simulink model "gov_modularised"  (R2020a)
settings: Solver=VariableStepAuto  StartTime=0.0  StopTime=10.0  RelTol=1e-3
values from neighbouring files (symbols this model uses):
  Amp = 0.1*10^6    (= 100000)    [main.m]
  Kd = 0.2*10^6    (= 200000)    [main.m]
  Ki = 0.2*10^6    (= 200000)    [main.m]
  Kp = 1*10^6    (= 1000000)    [main.m]
  sigma = 0.6    [main.m]
  Start = 1*10^6    (= 1000000)    [main.m]
  target_employment = 2700000    [main.m]
  Tf = 0.3    [main.m]
  Tg = 0.3    [main.m]
  Tpriv = 0.9    [main.m]
  Tpub = 0.9    [main.m]
  tx_firm = 0.3    [main.m]
  tx_priv = 0.4    [main.m]
  VAT = 0.07    [main.m]
libraries: simulink x1
settings Model: Creator=erlended  LastModifiedBy=erlended

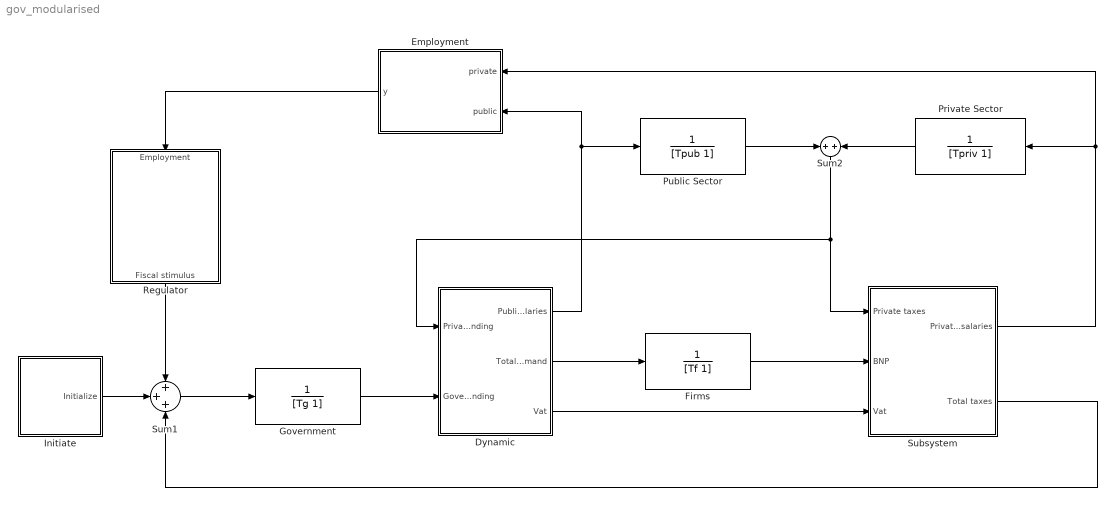
== system gov_modularised ==
  Dynamic : Subsystem
  Employment : Subsystem
  Firms : TransferFcn  Denominator=[Tf 1]
  Government : TransferFcn  Denominator=[Tg 1]
  Initiate : Subsystem
  Private Sector : TransferFcn  Denominator=[Tpriv 1]
  Public Sector : TransferFcn  Denominator=[Tpub 1]
  Regulator : Subsystem
  Subsystem : Subsystem
  Sum1 : Sum  Inputs=+++
  Sum2 : Sum  Inputs=+|+
  wires:
  Private Sector/1 -> Sum2/2
  Sum2/1 -> Subsystem/1(Private taxes), Dynamic/1(Private Spending)
  Public Sector/1 -> Sum2/1
  Sum1/1 -> Government/1
  Regulator/1(Fiscal stimulus) -> Sum1/1
  Employment/1(y) -> Regulator/1(Employment)
  Subsystem/2(Total taxes) -> Sum1/3
  Dynamic/1(Public salaries) -> Employment/2(public), Public Sector/1
  Government/1 -> Dynamic/2(Government spending)
  Dynamic/2(Total demand) -> Firms/1
  Subsystem/1(Private salaries) -> Employment/1(private), Private Sector/1
  Firms/1 -> Subsystem/2(BNP)
  Initiate/1(Initialize) -> Sum1/2
  Dynamic/3(Vat) -> Subsystem/3(Vat)

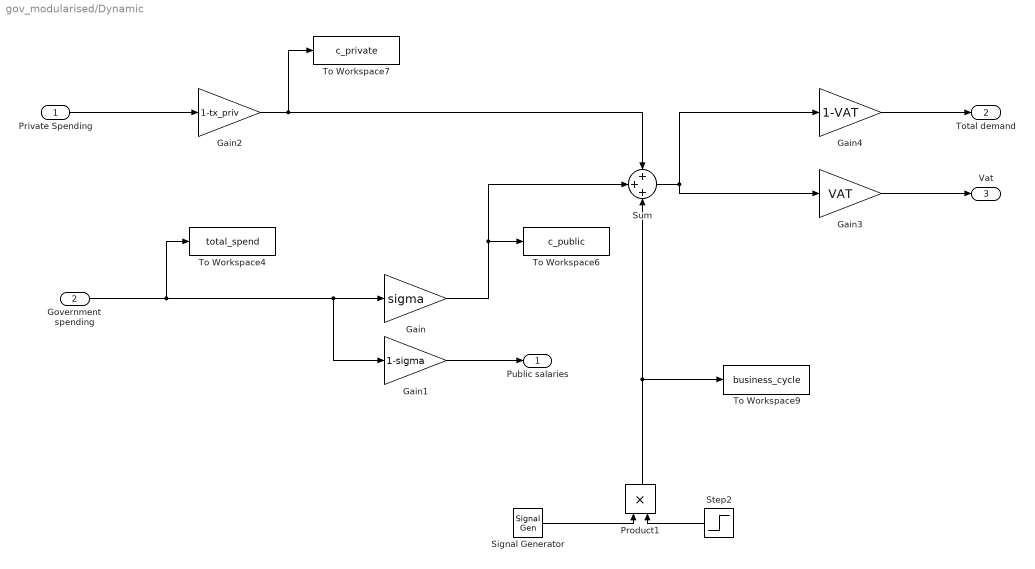
== system gov_modularised/Dynamic ==
  Private Spending : Inport
  Government spending : Inport  Port=2
  Gain : Gain  Gain=sigma
  Gain1 : Gain  Gain=1-sigma
  Gain2 : Gain  Gain=1-tx_priv
  Gain3 : Gain  Gain=VAT
  Gain4 : Gain  Gain=1-VAT
  Product1 : Product
  Signal Generator : SignalGenerator  Amplitude=Amp  Frequency=0.5  Units=rad/sec
  Step2 : Step  Time=30  SampleTime=0
  Sum : Sum  Inputs=+++
  To Workspace4 : ToWorkspace  VariableName=total_spend  SaveFormat=Timeseries  SampleTime=-1
  To Workspace6 : ToWorkspace  VariableName=c_public  SaveFormat=Timeseries  SampleTime=-1
  To Workspace7 : ToWorkspace  VariableName=c_private  SaveFormat=Timeseries  SampleTime=-1
  To Workspace9 : ToWorkspace  VariableName=business_cycle  SaveFormat=Timeseries  SampleTime=-1
  Public salaries : Outport
  Total demand : Outport  Port=2
  Vat : Outport  Port=3
  wires:
  Gain/1 -> To Workspace6/1, Sum/2
  Government spending/1 -> Gain/1, Gain1/1, To Workspace4/1
  Product1/1 -> Sum/3, To Workspace9/1
  Private Spending/1 -> Gain2/1
  Signal Generator/1 -> Product1/1
  Step2/1 -> Product1/2
  Sum/1 -> Gain3/1, Gain4/1
  Gain2/1 -> Sum/1, To Workspace7/1
  Gain1/1 -> Public salaries/1
  Gain4/1 -> Total demand/1
  Gain3/1 -> Vat/1

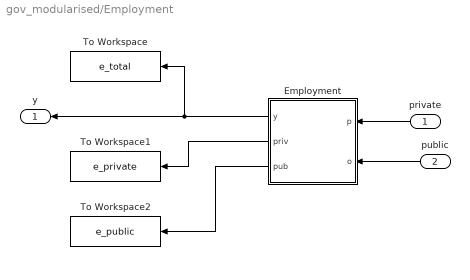
== system gov_modularised/Employment ==
  private : Inport
  public : Inport  Port=2
  Employment : MATLAB Function  TreatAsAtomicUnit=on
  To Workspace : ToWorkspace  VariableName=e_total  SaveFormat=Timeseries  SampleTime=-1
  To Workspace1 : ToWorkspace  VariableName=e_private  SaveFormat=Timeseries  SampleTime=-1
  To Workspace2 : ToWorkspace  VariableName=e_public  SaveFormat=Timeseries  SampleTime=-1
  y : Outport
  wires:
  Employment/2(priv) -> To Workspace1/1
  private/1 -> Employment/1(p)
  Employment/1(y) -> y/1, To Workspace/1
  Employment/3(pub) -> To Workspace2/1
  public/1 -> Employment/2(o)

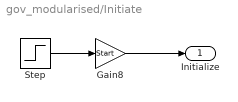
== system gov_modularised/Initiate ==
  Gain8 : Gain  Gain=Start
  Step : Step  Before=1  After=0  SampleTime=0
  Initialize : Outport
  wires:
  Step/1 -> Gain8/1
  Gain8/1 -> Initialize/1

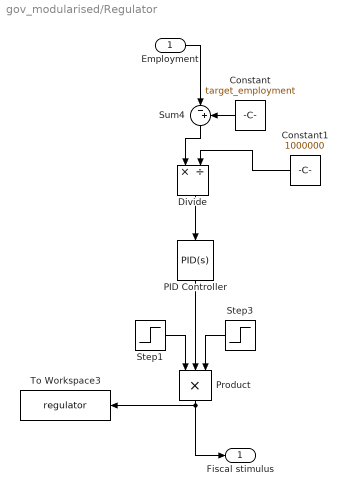
== system gov_modularised/Regulator ==
  Employment : Inport
  Constant : Constant  Value=target_employment
  Constant1 : Constant  Value=1000000
  Divide : Product  Inputs=*/
  PID Controller : simulink/Continuous/PID Controller  Controller=PID  Form=Parallel  TimeDomain=Continuous-time  UseExternalTs=off  SampleTime=-1  IntegratorMethod=Forward Euler  FilterMethod=Forward Euler  ControllerParametersSource=internal  P=Kp  I=Ki  D=Kd  UseFilter=on  N=1  TunerSelectOption=Transfer Function Based (PID Tuner App)  InitialConditionSource=internal  InitialConditionForIntegrator=0  InitialConditionForFilter=0  DifferentiatorICPrevScaledInput=0  ExternalReset=none  TrackingMode=off  Kt=1  LimitOutput=off  UpperSaturationLimit=inf  LowerSaturationLimit=-inf  LinearizeAsGain=on  AntiWindupMode=none  Kb=1  POutMin=[]  POutMax=[]  IOutMin=[]  IOutMax=[]  DOutMin=[]  DOutMax=[]  NOutMin=[]  NOutMax=[]  SumOutMin=[]  SumOutMax=[]  SaturationOutMin=[]  SaturationOutMax=[]  PParamMin=[]  PParamMax=[]  IParamMin=[]  IParamMax=[]  DParamMin=[]  DParamMax=[]  NParamMin=[]  NParamMax=[]  KbParamMin=[]  KbParamMax=[]  KtParamMin=[]  KtParamMax=[]  KbOutMin=[]  KbOutMax=[]  KtOutMin=[]  KtOutMax=[]  IntegratorOutMin=[]  IntegratorOutMax=[]  FilterOutMin=[]  FilterOutMax=[]  SumI1OutMin=[]  SumI1OutMax=[]  SumI2OutMin=[]  SumI2OutMax=[]  SumI3OutMin=[]  SumI3OutMax=[]  SumI4OutMin=[]  SumI4OutMax=[]  SumDOutMin=[]  SumDOutMax=[]  DifferentiatorOutMin=[]  DifferentiatorOutMax=[]  FilterDiffOutCoefMin=[]  FilterDiffOutCoefMax=[]  ReciprocalOutMin=[]  ReciprocalOutMax=[]  SumDenOutMin=[]  SumDenOutMax=[]  SumNumOutMin=[]  SumNumOutMax=[]  DivideOutMin=[]  DivideOutMax=[]  UdiffTsProdOutMin=[]  UdiffTsProdOutMax=[]  NTsProdOutMin=[]  NTsProdOutMax=[]  UintegralTsProdOutMin=[]  UintegralTsProdOutMax=[]  UngainTsProdOutMin=[]  UngainTsProdOutMax=[]  IntegratorContinuousStateAttributes=''  IntegratorStateMustResolveToSignalObject=off  IntegratorRTWStateStorageClass=Auto  FilterContinuousStateAttributes=''  FilterStateMustResolveToSignalObject=off  FilterRTWStateStorageClass=Auto  ParallelPVariant=InternalParameters  IdealPVariant=Disabled  IVariant=InternalParameters  DVariant=InternalParameters  IntegratorVariant=Continuous  SatVariant=Disabled  AWVariant=Passthrough  PCopyVariant=Disabled  TRVariant=Disabled  FdbkBlocksVariant=Forward  IdealPFdbkVariant=Disabled  SatFdbkVariant=Disabled  DerivativeFilterVariant=ContFilter  NVariant=InternalParameters  NCopyVariant=Disabled  FilterICVariant=InternalICsFilter  IntegratorICVariant=InternalICs  ExternalResetVariant=Disabled  TRSumVariant=Passthrough  SumFdbkVariant=Disabled  SumVariant=Sum_PID  TsampFilterVariant=InternalTs  TsampNgainVariant=Passthrough  TsampIntegralVariant=Passthrough
  Product : Product  Inputs=3
  Step1 : Step  SampleTime=0
  Step3 : Step  Time=50  Before=1  After=0  SampleTime=0
  Sum4 : Sum  Inputs=|-+
  To Workspace3 : ToWorkspace  VariableName=regulator  SaveFormat=Timeseries  SampleTime=-1
  Fiscal stimulus : Outport
  wires:
  Step1/1 -> Product/1
  PID Controller/1 -> Product/2
  Constant1/1 -> Divide/2
  Product/1 -> Fiscal stimulus/1, To Workspace3/1
  Divide/1 -> PID Controller/1
  Constant/1 -> Sum4/2
  Step3/1 -> Product/3
  Sum4/1 -> Divide/1
  Employment/1 -> Sum4/1

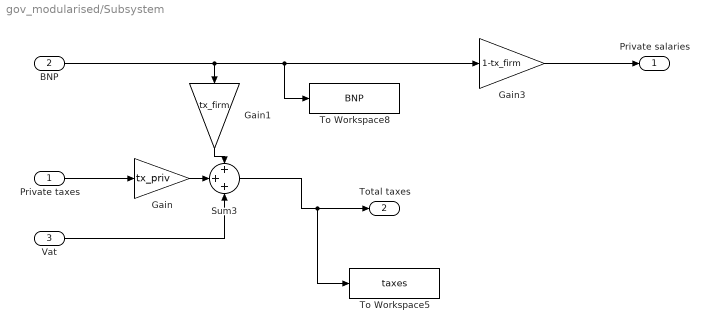
== system gov_modularised/Subsystem ==
  Private taxes : Inport
  BNP : Inport  Port=2
  Vat : Inport  Port=3
  Gain : Gain  Gain=tx_priv
  Gain1 : Gain  Gain=tx_firm
  Gain3 : Gain  Gain=1-tx_firm
  Sum3 : Sum  Inputs=+++
  To Workspace5 : ToWorkspace  VariableName=taxes  SaveFormat=Timeseries  SampleTime=-1
  To Workspace8 : ToWorkspace  VariableName=BNP  SaveFormat=Timeseries  SampleTime=-1
  Private salaries : Outport
  Total taxes : Outport  Port=2
  wires:
  BNP/1 -> Gain3/1, To Workspace8/1, Gain1/1
  Gain3/1 -> Private salaries/1
  Sum3/1 -> To Workspace5/1, Total taxes/1
  Private taxes/1 -> Gain/1
  Gain1/1 -> Sum3/1
  Gain/1 -> Sum3/2
  Vat/1 -> Sum3/3

== matlab function gov_modularised/Employment/Employment ==
  data: p input; o input; y output; priv output; pub output
function  [y, priv, pub]= fcn(p, o)
salary = 0.5; 

priv = p/(salary);
pub = o/(salary);
u = priv + pub;

y = u;
